simulink model "Bitwise"  (R2024b)
settings: Solver=VariableStepAuto  StartTime=0.0  StopTime=10.0  RelTol=1e-3
libraries: simulink x5
settings Model: Creator=abdal  LastModifiedBy=abdal

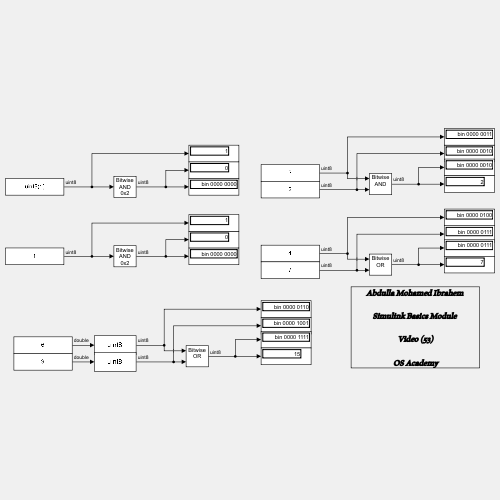
[thumbnail: Simulink's stored preview of the top-level diagram]
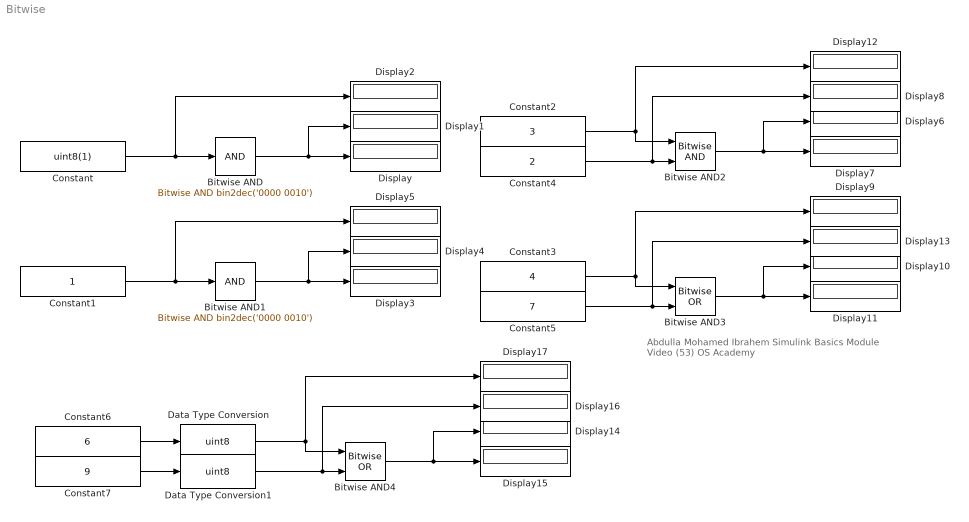
== system Bitwise ==
  note: Abdulla Mohamed Ibrahem
      | Simulink Basics Module
      | Video (53)
      | OS Academy
  Bitwise AND : simulink/Logic and Bit Operations/Bitwise Operator  logicop=AND  UseBitMask=on  BitMask=bin2dec('0000 0010')  BitMaskRealWorld=Stored Integer
      settings: LibrarySourceBlock=|
      | simulink/Quick Insert/Logic and Bit
      | Operations/Bitwise AND
  Bitwise AND1 : simulink/Logic and Bit Operations/Bitwise Operator  logicop=AND  UseBitMask=on  BitMask=bin2dec('0000 0010')  BitMaskRealWorld=Stored Integer
      settings: LibrarySourceBlock=|
      | simulink/Quick Insert/Logic and Bit
      | Operations/Bitwise AND
  Bitwise AND2 : simulink/Logic and Bit Operations/Bitwise Operator  logicop=AND  UseBitMask=off  NumInputPorts=2  BitMask=bin2dec('0000 0010')  BitMaskRealWorld=Stored Integer
      settings: LibrarySourceBlock=|
      | simulink/Quick Insert/Logic and Bit
      | Operations/Bitwise AND
  Bitwise AND3 : simulink/Logic and Bit Operations/Bitwise Operator  logicop=OR  UseBitMask=off  NumInputPorts=2  BitMask=bin2dec('0000 0010')  BitMaskRealWorld=Stored Integer
      settings: LibrarySourceBlock=|
      | simulink/Quick Insert/Logic and Bit
      | Operations/Bitwise AND
  Bitwise AND4 : simulink/Logic and Bit Operations/Bitwise Operator  logicop=OR  UseBitMask=off  NumInputPorts=2  BitMask=bin2dec('0000 0010')  BitMaskRealWorld=Stored Integer
      settings: LibrarySourceBlock=|
      | simulink/Quick Insert/Logic and Bit
      | Operations/Bitwise AND
  Constant : Constant  Value=uint8(1)
  Constant1 : Constant  OutDataTypeStr=uint8
  Constant2 : Constant  Value=3  OutDataTypeStr=uint8
  Constant3 : Constant  Value=4  OutDataTypeStr=uint8
  Constant4 : Constant  Value=2  OutDataTypeStr=uint8
  Constant5 : Constant  Value=7  OutDataTypeStr=uint8
  Constant6 : Constant  Value=6
  Constant7 : Constant  Value=9
  Data Type Conversion : DataTypeConversion  OutDataTypeStr=uint8  SaturateOnIntegerOverflow=off  RndMeth=Floor
  Data Type Conversion1 : DataTypeConversion  OutDataTypeStr=uint8  SaturateOnIntegerOverflow=off  RndMeth=Floor
  Display{,1..17} (18 alike) : Display
      Display settings: Format=binary (Stored Integer)
      Display10 settings: Format=binary (Stored Integer)
      Display12 settings: Format=binary (Stored Integer)
      Display13 settings: Format=binary (Stored Integer)
      Display14 settings: Format=binary (Stored Integer)
      Display16 settings: Format=binary (Stored Integer)
      Display17 settings: Format=binary (Stored Integer)
      Display3 settings: Format=binary (Stored Integer)
      Display6 settings: Format=binary (Stored Integer)
      Display8 settings: Format=binary (Stored Integer)
      Display9 settings: Format=binary (Stored Integer)
  wires:
  Constant/1 -> Display2/1, Bitwise AND/1
  Bitwise AND/1 -> Display1/1, Display/1
  Bitwise AND1/1 -> Display3/1, Display4/1
  Constant1/1 -> Bitwise AND1/1, Display5/1
  Constant2/1 -> Display12/1, Bitwise AND2/1
  Constant4/1 -> Display8/1, Bitwise AND2/2
  Bitwise AND2/1 -> Display7/1, Display6/1
  Bitwise AND3/1 -> Display10/1, Display11/1
  Constant5/1 -> Bitwise AND3/2, Display13/1
  Constant3/1 -> Bitwise AND3/1, Display9/1
  Constant6/1 -> Data Type Conversion/1
  Constant7/1 -> Data Type Conversion1/1
  Bitwise AND4/1 -> Display15/1, Display14/1
  Data Type Conversion/1 -> Display17/1, Bitwise AND4/1
  Data Type Conversion1/1 -> Display16/1, Bitwise AND4/2
